simulink model "robo1"  (R2024a)
settings: Solver=VariableStepAuto  StartTime=0.0  StopTime=10.0  RelTol=1e-3
settings Model: Creator=palan  LastModifiedBy=palan

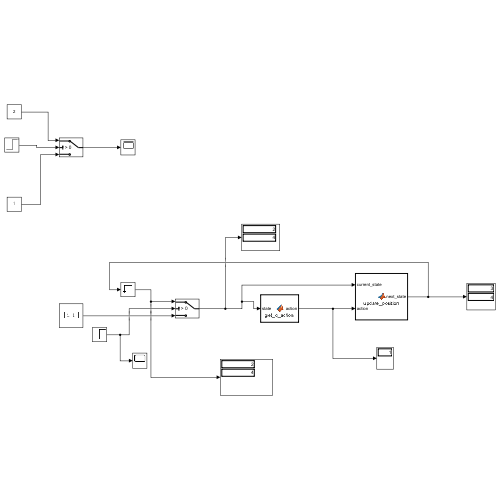
[thumbnail: Simulink's stored preview of the top-level diagram]
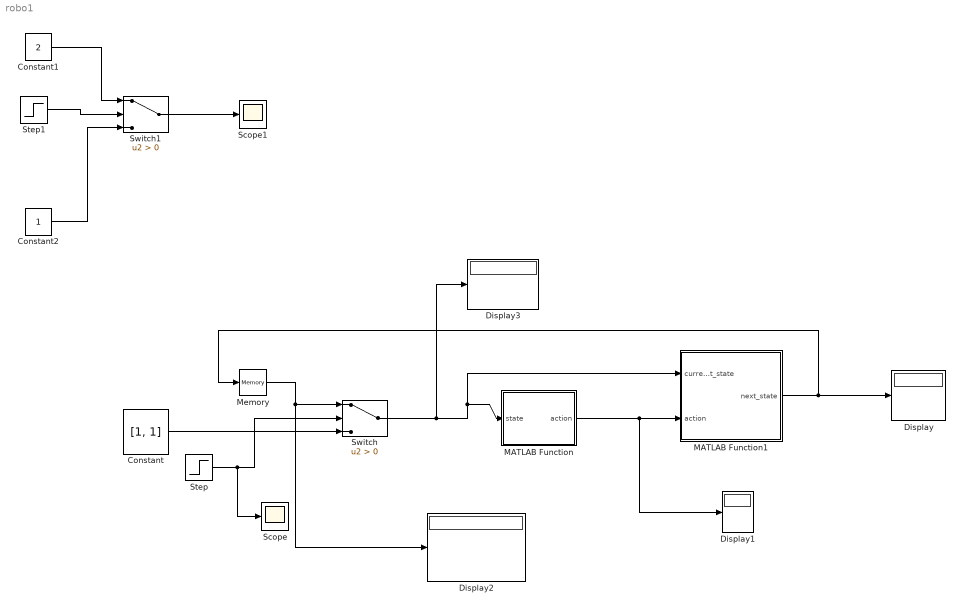
== system robo1 ==
  Constant : Constant  Value=[1, 1]
  Constant1 : Constant  Value=2
  Constant2 : Constant
  Display{,1..3} (4 alike) : Display
  MATLAB Function : MATLAB Function  TreatAsAtomicUnit=on
  MATLAB Function1 : MATLAB Function  TreatAsAtomicUnit=on
  Memory : Memory
  Scope : Scope
  Scope1 : Scope
  Step : Step  SampleTime=1
  Step1 : Step  SampleTime=0
  Switch : Switch  Criteria=u2 > Threshold  SaturateOnIntegerOverflow=off  InputSameDT=off
  Switch1 : Switch  Criteria=u2 > Threshold  SaturateOnIntegerOverflow=off  InputSameDT=off
  wires:
  MATLAB Function/1(action) -> Display1/1, MATLAB Function1/2(action)
  MATLAB Function1/1(next_state) -> Memory/1, Display/1
  Memory/1 -> Switch/1, Display2/1
  Switch/1 -> Display3/1, MATLAB Function1/1(current_state), MATLAB Function/1(state)
  Constant/1 -> Switch/3
  Step/1 -> Scope/1, Switch/2
  Step1/1 -> Switch1/2
  Constant2/1 -> Switch1/3
  Constant1/1 -> Switch1/1
  Switch1/1 -> Scope1/1

== matlab function robo1/MATLAB Function ==
  data: state input; action output
function action = get_q_action(state)
    persistent Q_table;
    
    % Load policy only once
    if isempty(Q_table)
        data = load('policy.mat');
        Q_table = data.policy; % Load Q-table
    end
    
    % Get the best action for the given state
    row = state(1);
    col = state(2);
    q_values = squeeze(Q_table(row, col, :)); % Extract Q-values for the state
    
    % Select action with the highest Q-value
    action = q_values;
end

== matlab function robo1/MATLAB Function1 ==
  data: current_state input; next_state output; action input
function next_state = update_position(current_state, action)
    % Define grid limits
    grid_size = [4, 4]; % 4x4 Grid World
    
    % Extract current position
    row = current_state(1);
    col = current_state(2);
    
    % Define action moves (same as Q-learning actions)
    moves = [-1 0;  % Up
             1 0;   % Down
             0 -1;  % Left
             0 1];  % Right
    
    % Get the movement offset from action
    move = moves(action + 1, :);
    
    % Compute next position
    new_row = min(max(row + move(1), 1), grid_size(1));  % Keep within bounds
    new_col = min(max(col + move(2), 1), grid_size(2));  % Keep within bounds
    
    % Return updated position
    next_state = [new_row; new_col];
end
